simulink model "ug"  (Simulink 8.9)
settings: Solver=ode4  StartTime=0.0  StopTime=1  MaxStep=1e-4  RelTol=1e-3
libraries: powerlib x21, simulink x7, powerlib_meascontrol x3
settings Model: Creator=tsukuyomi  LastModifiedBy=Sumanth Narkedamilli
settings DataIOCC: LimitDataPoints=off  SaveFormat=Dataset  SignalLoggingSaveFormat=Dataset
settings OptimizationCC: LifeSpan=auto
settings DebuggingCC: UnderspecifiedInitializationDetection=Simplified  MergeDetectMultiDrivingBlocksExec=error  FcnCallInpInsideContextMsg=error  StateNameClashWarn=none  SFUnexpectedBacktrackingDiag=error  SFNoUnconditionalDefaultTransitionDiag=error  SFExecutionAtInitializationDiag=warning
settings HardwareCC: ProdBitPerPointer=64  ProdBitPerSizeT=64  ProdBitPerPtrDiffT=64  ProdLargestAtomicFloat=Float  ProdIntDivRoundTo=Zero  ProdEndianess=LittleEndian  ProdWordSize=64  ProdHWDeviceType=Intel->x86-64 (Windows64)
settings ModelReferenceCC: PropagateSignalLabelsOutOfModel=on
settings GRTTargetCC: TargetLangStandard=C99 (ISO)  GeneratePreprocessorConditionals=Use local settings  CombineOutputUpdateFcns=on  GRTInterface=off
settings ConfigComp: CovMetricSettings=dwe  CovHtmlReporting=off  CovSaveCumulativeToWorkspaceVar=off  CovSaveSingleToWorkspaceVar=off  CovExternalEMLEnable=on

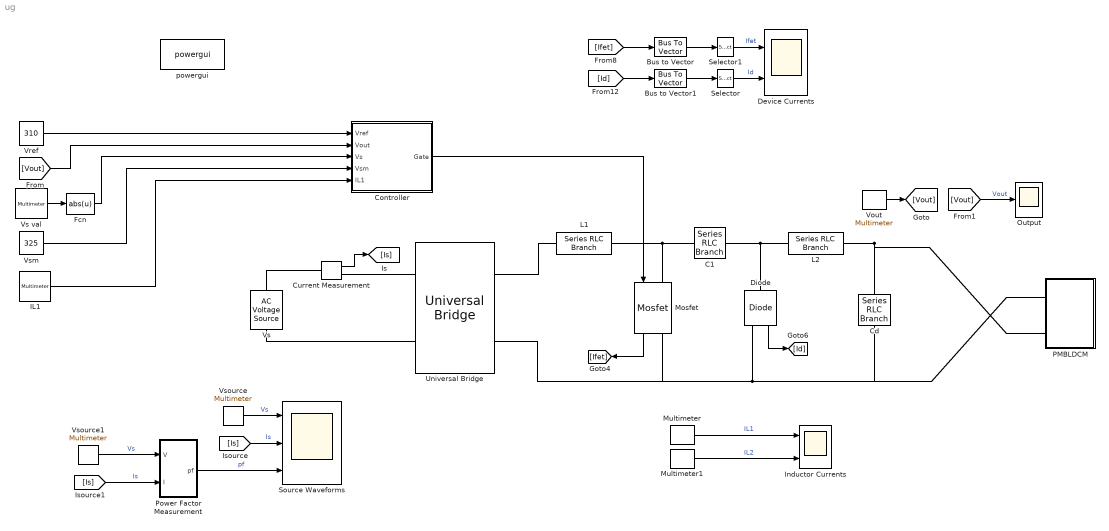
== system ug ==
  Bus to Vector : BusToVector
  Bus to Vector1 : BusToVector
  C1 : powerlib/Elements/Series RLC Branch  LConnTagsString=__new0  RConnTagsString=__new0  BranchType=C  Resistance=1e-4  Inductance=200e-6  SetiL0=off  InitialCurrent=0  Capacitance=0.36e-6  Setx0=off  InitialVoltage=40  Measurements=Branch voltage and current
  Cd : powerlib/Elements/Series RLC Branch  LConnTagsString=__new0  RConnTagsString=__new0  BranchType=C  Resistance=1e-3  Inductance=200e-6  SetiL0=off  InitialCurrent=0  Capacitance=1655e-6  Setx0=on  InitialVoltage=310  Measurements=Branch voltage
  Controller : Subsystem
  Current Measurement : powerlib/Measurements/Current Measurement  PhasorSimulation=off  OutputType=Complex  PSBequivalent=0
  Device Currents : Scope  NumInputPorts=2
  Diode : powerlib/Power Electronics/Diode  Ron=1e-3  Lon=0  Vf=0.7  IC=0  UseSnubber=off  Rs=inf  Cs=inf  Measurements=on
  Fcn : Fcn  Expr=abs(u)
  IL1 : powerlib/Measurements/Multimeter  PhasorSimulation=off  OutputType=Complex  sel=5  L=6  Gain=1  yselected={'Ib: L1'};  PSBOutputType=1  PSBequivalent=0  AxesSetting=[0,0.1,-100,100]  Display=0  SavedBlockNames=-11
  Inductor Currents : Scope  NumInputPorts=2
  L1 : powerlib/Elements/Series RLC Branch  LConnTagsString=__new0  RConnTagsString=__new0  BranchType=L  Resistance=1e-3  Inductance=5.03e-3  SetiL0=off  InitialCurrent=14  Capacitance=1e-6  Setx0=off  InitialVoltage=0  Measurements=Branch current
  L2 : powerlib/Elements/Series RLC Branch  LConnTagsString=__new0  RConnTagsString=__new0  BranchType=L  Resistance=1e-3  Inductance=0.58e-3  SetiL0=off  InitialCurrent=0  Capacitance=1e-6  Setx0=off  InitialVoltage=0  Measurements=Branch current
  Mosfet : powerlib/Power Electronics/Mosfet  Ron=1e-3  Lon=0  Rd=1e-3  Vfd=0.3  IC=0  Rs=1e6  Cs=inf  Measurements=on
  Multimeter : powerlib/Measurements/Multimeter  PhasorSimulation=off  OutputType=Complex  sel=5  L=6  Gain=1  yselected={'Ib: L1'};  PSBOutputType=1  PSBequivalent=0  AxesSetting=[0,0.1,-100,100]  Display=0  SavedBlockNames=-11
  Multimeter1 : powerlib/Measurements/Multimeter  PhasorSimulation=off  OutputType=Complex  sel=6  L=6  Gain=1  yselected={'Ib: L2'};  PSBOutputType=1  PSBequivalent=0  AxesSetting=[0,0.1,-100,100]  Display=0  SavedBlockNames=-11
  Output : Scope
  PMBLDCM : Subsystem
  Power Factor Measurement : Subsystem
  Selector : Selector  InputPortWidth=2  IndexOptions=Index vector (dialog)  Indices=1  OutputSizes=1
  Selector1 : Selector  InputPortWidth=2  IndexOptions=Index vector (dialog)  Indices=1  OutputSizes=1
  Source Waveforms : Scope  NumInputPorts=3
  Universal Bridge : powerlib/Power Electronics/Universal Bridge  Arms=2  SnubberResistance=1e5  SnubberCapacitance=inf  Device=Diodes  Ron=1e-2  Lon=0  ForwardVoltages="[  0  0  ]"  ForwardVoltage=0  GTOparameters=[ 10e-6 , 20e-6 ]  IGBTparameters=[ 1e-6 , 2e-6 ]  Measurements=None  Measurements_2=None  converterType=Rectifier
  Vout : powerlib/Measurements/Multimeter  PhasorSimulation=off  OutputType=Complex  sel=2  L=6  Gain=1  yselected={'Ub: Cd'};  PSBOutputType=1  PSBequivalent=0  AxesSetting=[0,0.1,-100,100]  Display=0  SavedBlockNames=-11
  Vref : Constant  Value=310
  Vs : powerlib/Electrical Sources/AC Voltage Source  Amplitude=325  Phase=0  Frequency=50  SampleTime=0  Measurements=Voltage  BusType=PV  Pref=10e3  Qref=0  Qmin=-inf  Qmax=+inf
  Vs val : powerlib/Measurements/Multimeter  PhasorSimulation=off  OutputType=Complex  sel=3  L=6  Gain=1  yselected={'Usrc: Vs'};  PSBOutputType=1  PSBequivalent=0  AxesSetting=[0,0.1,-100,100]  Display=0  SavedBlockNames=-11
  Vsm : Constant  Value=325
  Vsource : powerlib/Measurements/Multimeter  PhasorSimulation=off  OutputType=Complex  sel=3  L=6  Gain=1  yselected={'Usrc: Vs'};  PSBOutputType=1  PSBequivalent=0  AxesSetting=[0,0.1,-100,100]  Display=0  SavedBlockNames=-11
  Vsource1 : powerlib/Measurements/Multimeter  PhasorSimulation=off  OutputType=Complex  sel=3  L=6  Gain=1  yselected={'Usrc: Vs'};  PSBOutputType=1  PSBequivalent=0  AxesSetting=[0,0.1,-100,100]  Display=0  SavedBlockNames=-11
  powergui : powerlib/powergui  Priority=1  SimulationMode=Discrete  SampleTime=1e-6  frequency=60  Iterations=50  frequencyindice=0  Pbase=100e6  ErrMax=1e-4  UnitsV=kV  UnitsW=MW  buscounter=0  FunctionMessages=off  echomessages=off  EnableUseOfTLC=off  CurrentSourceSwitches=off  DisableSnubberDevices=off  DisableRonSwitches=off  DisableVfSwitches=off  DisplayEquations=off  SolverType=Tustin/Backward Euler (TBE)  Interpol=off  ExternalGateDelay=off  methode=off  Ts=100  x0status=blocks  SPID=on  SwTol=0  HookPort=off  RestoreLinks=warning  ResistiveCurrentMeasurement=off  Frange=[0:2:500]  Ylog=off  Xlog=on  ShowGrid=off  save=off  variable=ZData  structure=current  ZoomFFT=on  StartTime=0.5  cycles=20  DisplayStyle=1  fundamental=50  FreqAxis=off  MaxFrequency=1000  frequencyindicesteady=1  RmsSteady=1  display=off
  wires:
  Bus to Vector/1 -> Selector1/1
  Bus to Vector1/1 -> Selector/1
  Multimeter/1 -> Inductor Currents/1  "IL1"
  Multimeter1/1 -> Inductor Currents/2  "IL2"
  [Ifet] -> Bus to Vector/1
  [Id] -> Bus to Vector1/1
  Selector1/1 -> Device Currents/1  "Ifet"
  Mosfet/1 -> [Ifet]
  Selector/1 -> Device Currents/2  "Id"
  Diode/1 -> [Id]
  Vout/1 -> [Vout]
  Vref/1 -> Controller/1(Vref)
  IL1/1 -> Controller/5(IL1)
  [Vout] -> Controller/2(Vout)
  Vsm/1 -> Controller/4(Vsm)
  Current Measurement/1 -> [Is]
  Vsource/1 -> Source Waveforms/1  "Vs"
  [Is] -> Source Waveforms/2  "Is"
  [Vout] -> Output/1  "Vout"
  Vs val/1 -> Fcn/1
  Vsource1/1 -> Power Factor Measurement/1(V)  "Vs"
  [Is] -> Power Factor Measurement/2(I)  "Is"
  Power Factor Measurement/1(pf) -> Source Waveforms/3  "pf"
  Controller/1(Gate) -> Mosfet/1
  Fcn/1 -> Controller/3(Vs)
  connections:
  Diode/LConn1 -- L2/RConn1 -- C1/RConn1
  Mosfet/LConn1 -- L1/RConn1 -- C1/LConn1
  Cd/RConn1 -- L2/LConn1 -- PMBLDCM/LConn2
  Diode/RConn1 -- PMBLDCM/LConn1 -- Cd/LConn1 -- Mosfet/RConn1 -- Universal Bridge/RConn2
  L1/LConn1 -- Universal Bridge/RConn1
  Current Measurement/LConn1 -- Vs/RConn1
  Vs/LConn1 -- Universal Bridge/LConn2
  Current Measurement/RConn1 -- Universal Bridge/LConn1

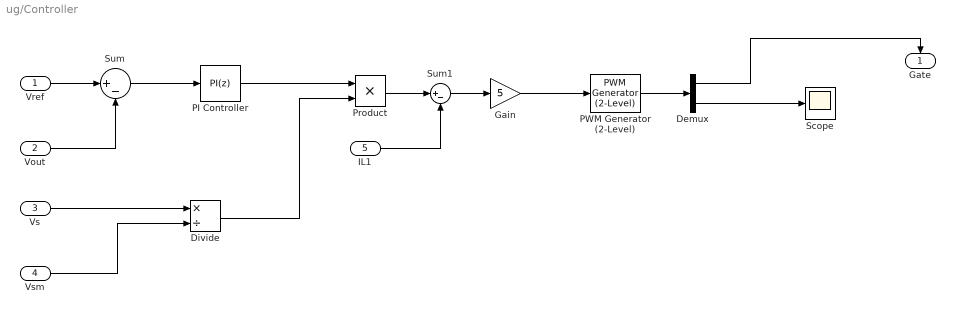
== system ug/Controller ==
  Vref : Inport
  Vout : Inport  Port=2
  Vs : Inport  Port=3
  Vsm : Inport  Port=4
  IL1 : Inport  Port=5
  Demux : Demux  Outputs=2
  Divide : Product  Inputs=*/
  Gain : Gain  Gain=5
  PI Controller : simulink/Continuous/PID Controller  Controller=PI  TimeDomain=Discrete-time  SampleTime=-1  IntegratorMethod=Forward Euler  FilterMethod=Forward Euler  Form=Parallel  UseFilter=on  ControllerParametersSource=internal  P=0.12  I=1.85  D=0  N=100  InitialConditionSource=internal  InitialConditionForIntegrator=0  InitialConditionForFilter=0  ExternalReset=none  LimitOutput=off  UpperSaturationLimit=inf  LowerSaturationLimit=-inf  LinearizeAsGain=on  AntiWindupMode=none  Kb=1  TrackingMode=off  Kt=1  PParamMin=[]  PParamMax=[]  IParamMin=[]  IParamMax=[]  DParamMin=[]  DParamMax=[]  NParamMin=[]  NParamMax=[]  KbParamMin=[]  KbParamMax=[]  KtParamMin=[]  KtParamMax=[]  POutMin=[]  POutMax=[]  IOutMin=[]  IOutMax=[]  DOutMin=[]  DOutMax=[]  NOutMin=[]  NOutMax=[]  KbOutMin=[]  KbOutMax=[]  KtOutMin=[]  KtOutMax=[]  IntegratorOutMin=[]  IntegratorOutMax=[]  FilterOutMin=[]  FilterOutMax=[]  SumOutMin=[]  SumOutMax=[]  SumI1OutMin=[]  SumI1OutMax=[]  SumI2OutMin=[]  SumI2OutMax=[]  SumI3OutMin=[]  SumI3OutMax=[]  SumDOutMin=[]  SumDOutMax=[]  SaturationOutMin=[]  SaturationOutMax=[]  IntegratorContinuousStateAttributes=''  IntegratorStateMustResolveToSignalObject=off  IntegratorRTWStateStorageClass=Auto  FilterContinuousStateAttributes=''  FilterStateMustResolveToSignalObject=off  FilterRTWStateStorageClass=Auto  DifferentiatorICPrevScaledInput=0  DifferentiatorOutMin=[]  DifferentiatorOutMax=[]  InitialConditionSetting=State (most efficient)
  PWM Generator (2-Level) : powerlib_meascontrol/Pulse & Signal Generators/PWM Generator (2-Level)  ModulatorType=Single-phase half-bridge (2 pulses)  ModulatorMode=Unsynchronized  Fc=40e3  Pc=0  nF=27  MinMax="[ 0  1 ]"  SamplingTechnique=Natural  ModulatingSignals=off  m=0.8  Freq=60  Phase=0  Ts=0  ShowCarrierOutport=off
      settings: SourceProductName=Simscape Power Systems
  Product : Product
  Scope : Scope
  Sum : Sum  Inputs=|+-
  Sum1 : Sum  Inputs=|+-
  Gate : Outport
  wires:
  Sum/1 -> PI Controller/1
  Vs/1 -> Divide/1
  PWM Generator (2-Level)/1 -> Demux/1
  Demux/1 -> Gate/1
  Product/1 -> Sum1/1
  Demux/2 -> Scope/1
  Divide/1 -> Product/2
  PI Controller/1 -> Product/1
  Vout/1 -> Sum/2
  Vsm/1 -> Divide/2
  Vref/1 -> Sum/1
  IL1/1 -> Sum1/2
  Sum1/1 -> Gain/1
  Gain/1 -> PWM Generator (2-Level)/1

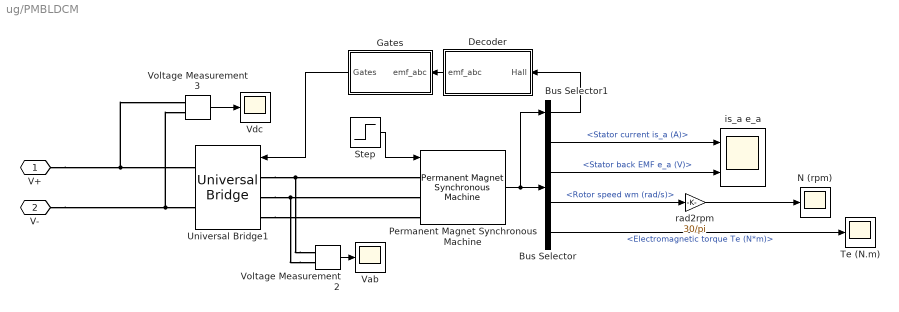
== system ug/PMBLDCM ==
  Bus Selector : BusSelector  OutputSignals=Stator current is_a (A),Stator back EMF e_a (V),Rotor speed wm (rad/s),Electromagnetic torque Te (N*m)
  Bus Selector1 : BusSelector  OutputSignals=Hall effect signal h_a,Hall effect signal h_b,Hall effect signal h_c  OutputAsBus=on
  Decoder : Subsystem
  Gates : Subsystem
  N (rpm) : Scope
  Permanent Magnet Synchronous Machine : powerlib/Machines/Permanent Magnet Synchronous Machine  NbPhases=3  FluxDistribution=Trapezoidal  RotorType=Round  MechanicalLoad=Torque Tm  PresetModel=No  ShowDetailedParameters=on  MeasurementBus=off  Resistance=1.09  Inductance=0.00765  dqInductances=[8.5e-3, 8.5e-3]  La=0.000835  MachineConstant=Flux linkage established by magnets (V.s)  Flux=0.1225  VoltageCst=51.3127  TorqueCst=0.49  Flat=120  Mechanical=[0.00014 0 2]  PolePairs=4  InitialConditions=[0,0, 0,0]  InitialConditions5ph=[0 0 0 0 0 0]  TsPowergui=0  TsBlock=-1  RefAngle=90 degrees behind phase A axis (modified Park)
      settings: SourceProductName=Simscape Power Systems
  Step : Step  Time=0.1  SampleTime=0
  Te (N.m) : Scope
  Universal Bridge1 : powerlib/Power Electronics/Universal Bridge  Arms=3  SnubberResistance=5000  SnubberCapacitance=1e-6  Device=MOSFET / Diodes  Ron=1e-3  Lon=0  ForwardVoltages="[  0  0  ]"  ForwardVoltage=0  GTOparameters=[ 10e-6 , 20e-6 ]  IGBTparameters=[ 1e-6 , 2e-6 ]  Measurements=None  Measurements_2=None  converterType=Rectifier
  Vab : Scope
  Vdc : Scope
  Voltage Measurement2 : powerlib/Measurements/Voltage Measurement  PhasorSimulation=off  OutputType=Complex  PSBequivalent=0
  Voltage Measurement3 : powerlib/Measurements/Voltage Measurement  PhasorSimulation=off  OutputType=Complex  PSBequivalent=0
  is_a e_a : Scope  NumInputPorts=2
  rad2rpm : Gain  Gain=30/pi
  V+ : PMIOPort  Port=1  Side=Left
  V- : PMIOPort  Port=2  Side=Left
  wires:
  Bus Selector1/1 -> Decoder/1("Hall ")
  rad2rpm/1 -> N (rpm)/1
  Bus Selector/2 -> is_a e_a/2  "<Stator back EMF e_a (V)>"
  Voltage Measurement3/1 -> Vdc/1
  Permanent Magnet Synchronous Machine/1 -> Bus Selector/1, Bus Selector1/1
  Gates/1(Gates) -> Universal Bridge1/1
  Bus Selector/4 -> Te (N.m)/1  "<Electromagnetic torque Te (N*m)>"
  Bus Selector/3 -> rad2rpm/1  "<Rotor speed wm (rad/s)>"
  Decoder/1(emf_abc) -> Gates/1("emf_abc ")
  Voltage Measurement2/1 -> Vab/1
  Step/1 -> Permanent Magnet Synchronous Machine/1
  Bus Selector/1 -> is_a e_a/1  "<Stator current is_a (A)>"
  connections:
  V-/RConn1 -- Voltage Measurement3/LConn2 -- Universal Bridge1/RConn2
  Voltage Measurement2/LConn2 -- Universal Bridge1/LConn2 -- Permanent Magnet Synchronous Machine/LConn2
  Universal Bridge1/LConn3 -- Permanent Magnet Synchronous Machine/LConn3
  Voltage Measurement2/LConn1 -- Universal Bridge1/LConn1 -- Permanent Magnet Synchronous Machine/LConn1
  V+/RConn1 -- Voltage Measurement3/LConn1 -- Universal Bridge1/RConn1

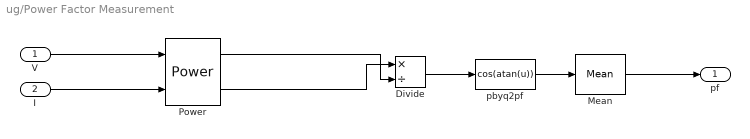
== system ug/Power Factor Measurement ==
  V : Inport
  I : Inport  Port=2
  Divide : Product  Inputs=*/
  Mean : powerlib_meascontrol/Measurements/Mean  Freq=50  Vinit=0  Ts=0
  Power : powerlib_meascontrol/Measurements/Power  Freq=50  Vinit=[1, 0]  Iinit=[1, 0]  Ts=0
      settings: SourceProductName=Simscape Power Systems
  pbyq2pf : Fcn  Expr=cos(atan(u))
  pf : Outport
  wires:
  Power/2 -> Divide/1
  Divide/1 -> pbyq2pf/1
  Power/1 -> Divide/2
  pbyq2pf/1 -> Mean/1
  V/1 -> Power/1
  I/1 -> Power/2
  Mean/1 -> pf/1

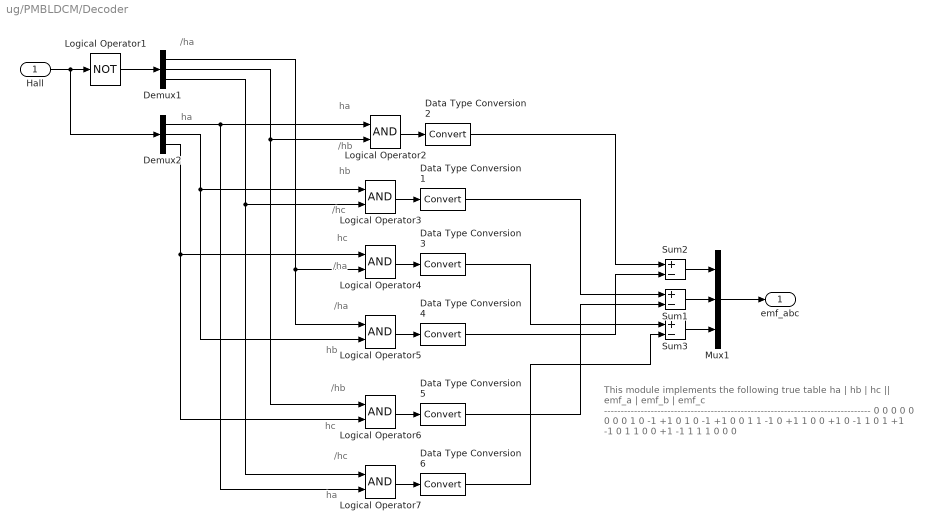
== system ug/PMBLDCM/Decoder ==
  note: /ha
  note: ha
  note: ha
  note: /hb
  note: hb
  note: /hc
  note: hc
  note: /ha
  note: /ha
  note: hb
  note: /hb
  note: hc
  note: /hc
  note: ha
  note: This module implements the following true table
      |
      |    ha   |   hb   |   hc   ||   emf_a   |   emf_b   |   emf_c
      |     --------------------------------------------------------------------------------
      | 0          0         0          0               0               0
      | 0          0         1          0               -1              +1
      | 0          1         0          -1              +1                0
      | 0          1         1          -1               0               +1
      | 1          0         0         +1               0               -1
      | 1          0         1         +1              -1                0
      | 1          1         0          0              +1               -1
      | 1          1         1          0               0                0
  "Hall " : Inport
  Data Type Conversion{1..6} (6 alike) : DataTypeConversion
  Demux1 : Demux  Outputs=3
  Demux2 : Demux  Outputs=3
  Logical Operator1 : Logic  Operator=NOT  AllPortsSameDT=off  OutDataTypeStr=boolean
  Logical Operator{2..7} (6 alike) : Logic  AllPortsSameDT=off  OutDataTypeStr=boolean
  Mux1 : Mux  Inputs=3
  Sum1 : Sum  Inputs=+-  OutDataTypeStr=double
  Sum2 : Sum  Inputs=+-  OutDataTypeStr=double
  Sum3 : Sum  Inputs=+-  OutDataTypeStr=double
  emf_abc : Outport
  wires:
  "Hall "/1 -> Logical Operator1/1, Demux2/1
  Logical Operator1/1 -> Demux1/1
  Demux2/3 -> Logical Operator4/1, Logical Operator6/2
  Demux2/2 -> Logical Operator3/1, Logical Operator5/2
  Demux2/1 -> Logical Operator2/1, Logical Operator7/2
  Demux1/3 -> Logical Operator3/2, Logical Operator7/1
  Demux1/2 -> Logical Operator2/2, Logical Operator6/1
  Demux1/1 -> Logical Operator4/2, Logical Operator5/1
  Logical Operator2/1 -> Data Type Conversion2/1
  Sum2/1 -> Mux1/1
  Sum1/1 -> Mux1/2
  Sum3/1 -> Mux1/3
  Mux1/1 -> emf_abc/1
  Logical Operator3/1 -> Data Type Conversion1/1
  Logical Operator4/1 -> Data Type Conversion3/1
  Logical Operator5/1 -> Data Type Conversion4/1
  Logical Operator6/1 -> Data Type Conversion5/1
  Logical Operator7/1 -> Data Type Conversion6/1
  Data Type Conversion2/1 -> Sum2/1
  Data Type Conversion4/1 -> Sum2/2
  Data Type Conversion1/1 -> Sum1/1
  Data Type Conversion5/1 -> Sum1/2
  Data Type Conversion3/1 -> Sum3/1
  Data Type Conversion6/1 -> Sum3/2

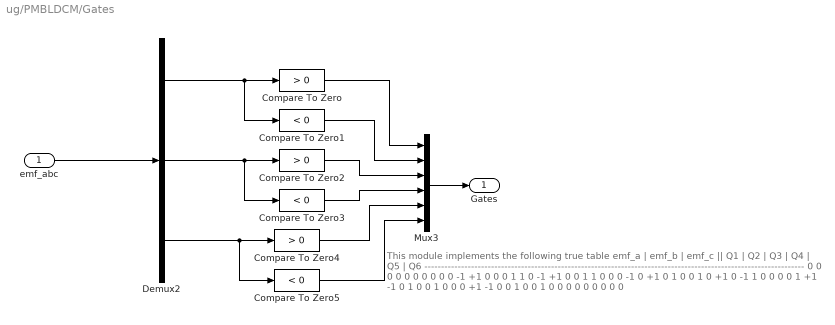
== system ug/PMBLDCM/Gates ==
  note: This module implements the following true table
      |
      |    emf_a   |   emf_b   |   emf_c   ||   Q1   |   Q2   |   Q3   |   Q4   |   Q5   |   Q6
      |     ------------------------------------------------------------------------------------------------------------------
      |       0              0                0            0          0          0           0        0        0
      |       0               -1              +1          0          0          0           1        1        0
      |     -1              +1                0          0          1          1           0        0        0
      |     -1               0               +1          0          1         0           0        1        0
      |    +1               0                -1          1          0          0           0        0        1
      |    +1              -1                0           1          0          0           1        0        0
      |      0              +1               -1           0          0          1           0        0        1
      |     0              0                0             0          0          0           0        0        0
  "emf_abc " : Inport
  Compare To Zero : simulink/Logic and Bit Operations/Compare To Zero  relop=>  OutDataTypeStr=boolean  ZeroCross=off
  Compare To Zero1 : simulink/Logic and Bit Operations/Compare To Zero  relop=<  OutDataTypeStr=boolean  ZeroCross=off
  Compare To Zero2 : simulink/Logic and Bit Operations/Compare To Zero  relop=>  OutDataTypeStr=boolean  ZeroCross=off
  Compare To Zero3 : simulink/Logic and Bit Operations/Compare To Zero  relop=<  OutDataTypeStr=boolean  ZeroCross=off
  Compare To Zero4 : simulink/Logic and Bit Operations/Compare To Zero  relop=>  OutDataTypeStr=boolean  ZeroCross=off
  Compare To Zero5 : simulink/Logic and Bit Operations/Compare To Zero  relop=<  OutDataTypeStr=boolean  ZeroCross=off
  Demux2 : Demux  Outputs=3
  Mux3 : Mux  Inputs=6
  Gates : Outport
  wires:
  "emf_abc "/1 -> Demux2/1
  Mux3/1 -> Gates/1
  Demux2/1 -> Compare To Zero/1, Compare To Zero1/1
  Demux2/2 -> Compare To Zero2/1, Compare To Zero3/1
  Demux2/3 -> Compare To Zero4/1, Compare To Zero5/1
  Compare To Zero/1 -> Mux3/1
  Compare To Zero1/1 -> Mux3/2
  Compare To Zero2/1 -> Mux3/3
  Compare To Zero3/1 -> Mux3/4
  Compare To Zero4/1 -> Mux3/5
  Compare To Zero5/1 -> Mux3/6
